simulink model "DDS_Stream_Ex1"  (R2023a)
settings: Solver=VariableStepAuto  StartTime=0.0  StopTime=0.01  RelTol=1e-3
undefined symbols (not defined in the file): None, S, vsva2197, xcvc1902
libraries: aieDSP x1, dspsigops x1, vmcUtilities x1
settings Model: Creator=sdegala  LastModifiedBy=robg
settings ModelReferenceCC: EnableRefExpFcnMdlSchedulingChecks=on

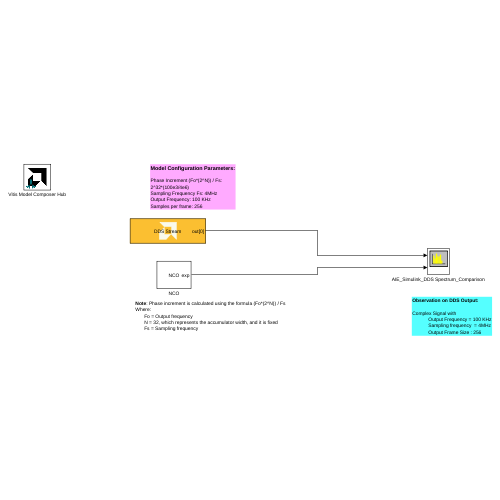
[thumbnail: Simulink's stored preview of the top-level diagram]
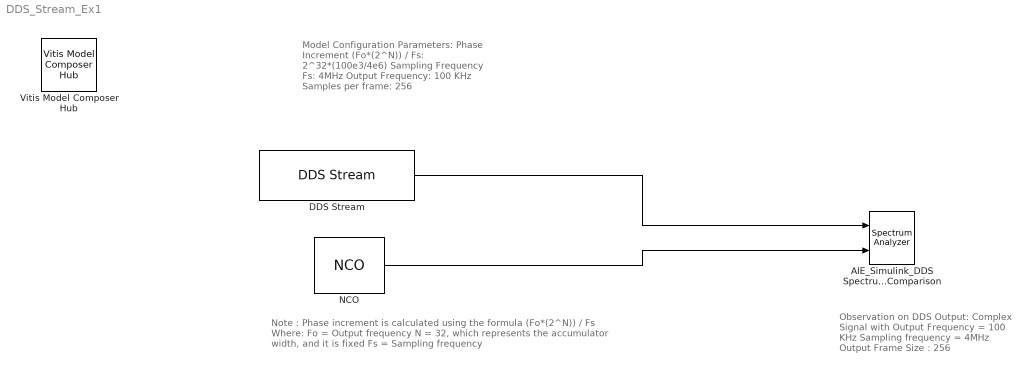
== system DDS_Stream_Ex1 ==
  note: Model Configuration Parameters:
      |
      | Phase Increment (Fo*(2^N)) / Fs:
      | 2^32*(100e3/4e6)
      | Sampling Frequency Fs: 4MHz
      | Output Frequency: 100 KHz
      | Samples per frame: 256
  note: Note : Phase increment is calculated using the formula (Fo*(2^N)) / Fs
      | Where:
      | Fo = Output frequency
      | N = 32, which represents the accumulator width, and it is fixed
      | Fs = Sampling frequency
  note: Observation on DDS Output:
      |
      | Complex Signal with
      | Output Frequency = 100 KHz
      | Sampling frequency = 4MHz
      | Output Frame Size : 256
  AIE_Simulink_DDS Spectrum_Comparison : SpectrumAnalyzer  NumInputPorts=2  AveragingMethod=Exponential  ShowLegend=on  ChannelNames="[\"\"]"  DefaultConfigurationName=spbscopes.SpectrumAnalyzerBlockCfg
  DDS Stream : aieDSP/DDS Stream  data_type=cfloat  output_window_size=256  ssr=1  USE_PHASE_RELOAD=off  phase_increment=1.0737e+08  initial_phase_offset=0  rnd_mode=Round to positive infinity  sat_mode=0-None  vmc_sample_time=1/4e6  AIE_VARIANT=1  blockJsonConstraints=[]  blockJsonConstraintsInternal=[]  spec=vmc_stream_dds.json  SerializedMaskParamNames=[]  SerializedMaskParamValues=[]  SerializedMaskParamVisibilities=[]  block_type=DDS Stream  SerializedMaskParamDataypes=typename|uint|uint|bool|uint|uint|uint|uint|double|uint  SerializedMaskParamEnumStrArr=0|0|0|0|0|0|Floor,Ceiling,Round to positive infinity,Round to negative infinity,Round symmetrical to infinity,Round symmetrical to zero,Round convergent to even,Round convergent to odd|0-None,1-Asymmetric,3-Symmetric|0|0  SerializedMaskParamEnumValArr=0|0|0|0|0|0|0,1,2,3,4,5,6,7|0,1,3|0|0  SerializedMaskParamVectorArr=0|0|0|0|0|0|0|0|0|0
  NCO : dspsigops/NCO  AccIncSrc=Specify via dialog  AccInc=1.0737e+08  PhaseOffsetSrc=Specify via dialog  PhaseOffset=0  AccumWL=32  HasDither=off  DitherWL=4  PNgeneratorLength=19  HasPhaseQuantizer=on  TableDepth=16  HasOutputPhaseError=off  Formula=Complex exponential  DataType=single  OutputWL=16  OutputFL=14  CompMethod=Table lookup (no interpolation)  SampleTime=1/4e6  SamplesPerFrame=256  OutputFrames=off
  Vitis Model Composer Hub : vmcUtilities/Vitis Model Composer Hub  Tag=genX  CodeGeneration=off  StartColumn=1  NumberOfColumns=1  TargetDirectory=./code  exportDesign=off  analyzeDesign=off  validateDesignOnHw=off  ExportType=AI Engines  IpVendor=xilinx.com  IpLibrary=hls  IpVersion=1.0  IpHWLanguage=Verilog  AieCompilerOptions={}  AieSimulatorOptions={}  CreateTestbench=off  TestbenchStackSize=10  RunRtlSim=off  RunCSim=off  RunAieSim=off  AieSimTimeout=50000  RunAieSimProfiling=off  LaunchVitisAnalyzer=off  PlotOutput=off  RunX86Sim=off  X86SimTimeout=10  GenHwImage=off  GenLibadfXo=off  GenHwValidationCode=off  PlatformType=Not Specified  HwSystemType=Baremetal  HwValidationTarget=hw  ProjDevice=xcvc1902-vsva2197-1LP-e-S  ProjDevicePart=xcvc1902-vsva2197-1LP-e-S  AIEType=AIE  SamplePeriod=-1  ClockFrequency=200  DataPathParallelism=1  xilinxfamily=versalaicore  part=xcvc1902  speed=-1LP-e-S  package=vsva2197  directory=./netlist  testbench=off  incr_netlist=off  synthesis_tool=Vivado  clock_wrapper=Clock Enables  dbl_ovrd=According to Block Masks  dcm_input_clock_period=10  sysclk_period=10  simulink_period=1  eval_field=0  LogFileName=''  NThreads=4
  wires:
  DDS Stream/1 -> AIE_Simulink_DDS Spectrum_Comparison/1
  NCO/1 -> AIE_Simulink_DDS Spectrum_Comparison/2
